simulink model "main"  (R2024b)
settings: Solver=VariableStepAuto  StartTime=0.0  StopTime=10.0  RelTol=1e-3
settings Model: Creator=tkhamvilai  LastModifiedBy=tkhamvilai

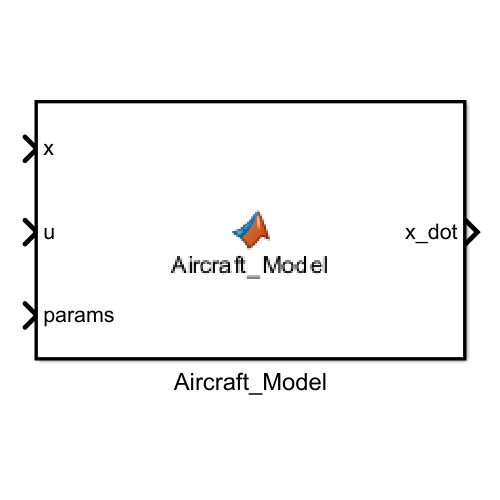
[thumbnail: Simulink's stored preview of the top-level diagram]
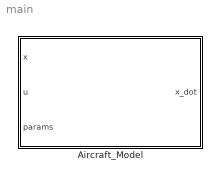
== system main ==
  Aircraft_Model : MATLAB Function  TreatAsAtomicUnit=on

== matlab function main/Aircraft_Model ==
  data: x input; u input; x_dot output; params input
function x_dot = Aircraft_Model(x,u,params)

x_dot = x + u;
